simulink model "SIMUclase2CI"  (R2022a)
settings: Solver=VariableStepAuto  StartTime=0.0  StopTime=10.0  RelTol=1e-3
values from neighbouring files (symbols this model uses):
  c = [1 1 0 1 1 1 1 1 1 1]    [BCD_entrenar.m]    (also in Clase2CI.m = 0.5; net1.mat)
  in = 3    [Clase2CI.m]
  k = 1    [Clase2CI.m]
  m = 0.25    [Clase2CI.m]
settings Model: Creator=meliodassama  LastModifiedBy=meliodassama

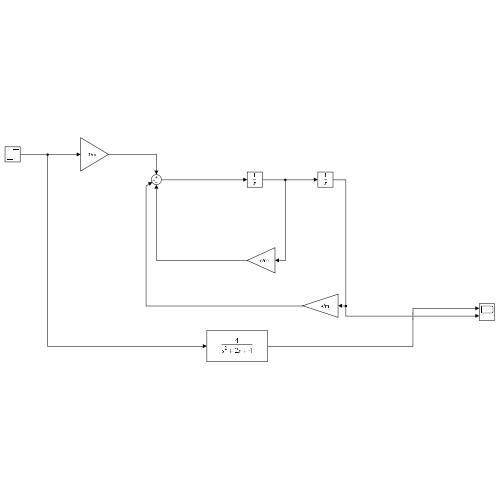
[thumbnail: Simulink's stored preview of the top-level diagram]
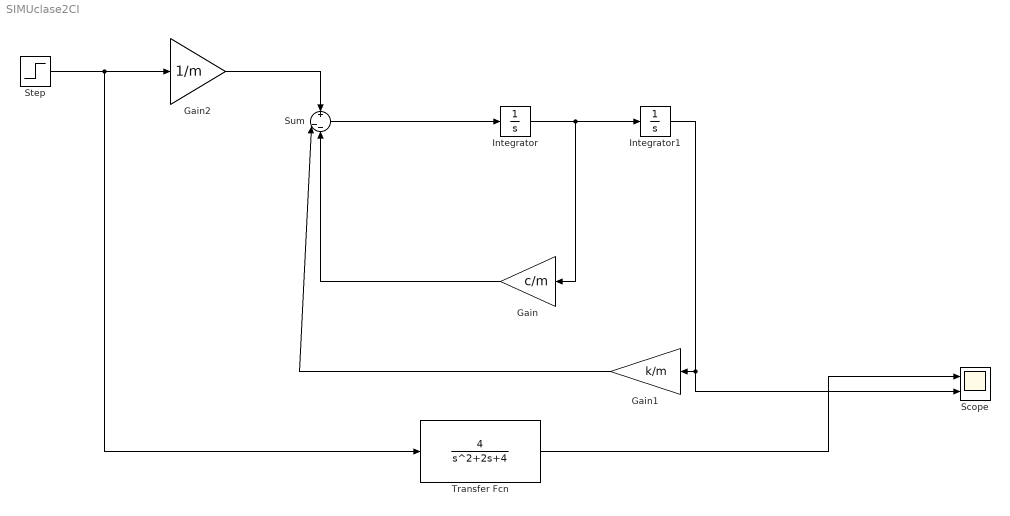
== system SIMUclase2CI ==
  Gain : Gain  Gain=c/m
  Gain1 : Gain  Gain=k/m
  Gain2 : Gain  Gain=1/m
  Integrator : Integrator
  Integrator1 : Integrator
  Scope : Scope  NumInputPorts=2
  Step : Step  Time=0  After=in  SampleTime=0
  Sum : Sum  Inputs=+|--
  Transfer Fcn : TransferFcn  Numerator=4  Denominator=[1 2 4]
  wires:
  Integrator/1 -> Gain/1, Integrator1/1
  Integrator1/1 -> Scope/2, Gain1/1
  Gain/1 -> Sum/3
  Gain1/1 -> Sum/2
  Sum/1 -> Integrator/1
  Gain2/1 -> Sum/1
  Step/1 -> Transfer Fcn/1, Gain2/1
  Transfer Fcn/1 -> Scope/1
